simulink model "P90s"  (R2015b)
settings: Solver=VariableStepAuto  StartTime=0.0  StopTime=3  RelTol=1e-3
settings Model: Creator=xmax1946  LastModifiedBy=xmax1946

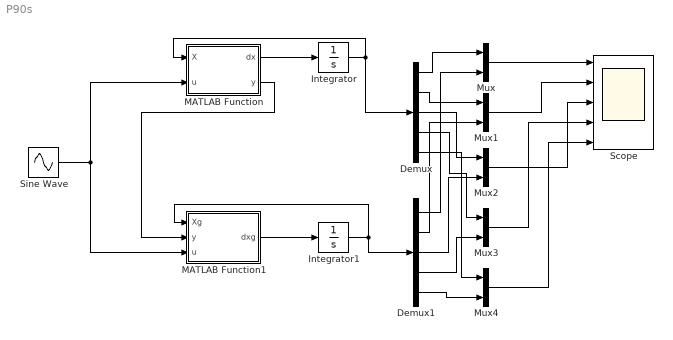
== system P90s ==
  Demux : Demux  Outputs=5
  Demux1 : Demux  Outputs=5
  Integrator : Integrator  InitialCondition=[1;1;1;1;1]
  Integrator1 : Integrator  InitialCondition=[pi;pi;pi;pi;pi]
  MATLAB Function : MATLAB Function  TreatAsAtomicUnit=on
  MATLAB Function1 : MATLAB Function  TreatAsAtomicUnit=on
  Mux{,1..4} (5 alike) : Mux  Inputs=2
  Scope : Scope  NumInputPorts=5
  Sine Wave : Sin  Amplitude=10  SampleTime=0
  wires:
  MATLAB Function/1(dx) -> Integrator/1
  MATLAB Function1/1(dxg) -> Integrator1/1
  Integrator/1 -> MATLAB Function/1(X), Demux/1
  MATLAB Function/2(y) -> MATLAB Function1/2(y)
  Integrator1/1 -> MATLAB Function1/1(Xg), Demux1/1
  Demux/1 -> Mux/1
  Demux1/1 -> Mux/2
  Demux/2 -> Mux1/1
  Demux1/2 -> Mux1/2
  Mux/1 -> Scope/1
  Mux1/1 -> Scope/2
  Sine Wave/1 -> MATLAB Function1/3(u), MATLAB Function/2(u)
  Demux/3 -> Mux2/1
  Demux1/3 -> Mux2/2
  Demux/4 -> Mux3/1
  Demux1/4 -> Mux3/2
  Demux/5 -> Mux4/1
  Demux1/5 -> Mux4/2
  Mux2/1 -> Scope/3
  Mux3/1 -> Scope/4
  Mux4/1 -> Scope/5

== matlab function P90s/MATLAB Function1 ==
  data: Xg input; y input; u input; dxg output
function dxg =fcn(Xg,y,u)
A=[0,-1,0,0,-4;0,0,1,0,1;0,1,0,0,2;-2,1,0,-2,4;0,0,0,0,-2];
B=[0;1;0;0;0];
C=[1,0,0,0,0];
L=[10;-32;-71;0;-1];

dxg=A*Xg+B*u+L*(y-C*Xg);

== matlab function P90s/MATLAB Function ==
  data: dx output; X input; y output; u input
function [dx,y]=fcn(X,u)
A=[0,-1,0,0,-4;0,0,1,0,1;0,1,0,0,2;-2,1,0,-2,4;0,0,0,0,-2];
B=[0;1;0;0;0];
C=[1,0,0,0,0];

dx=A*X+B*u;
y=C*X;
